simulink model "chap6_4sim"  (Simulink 3.00)
settings: Solver=ode45  StartTime=0.0  StopTime=3  RelTol=1e-3
settings Model: SaveTime=off  SaveOutput=off  Decimation=100  LastModifiedBy=liu

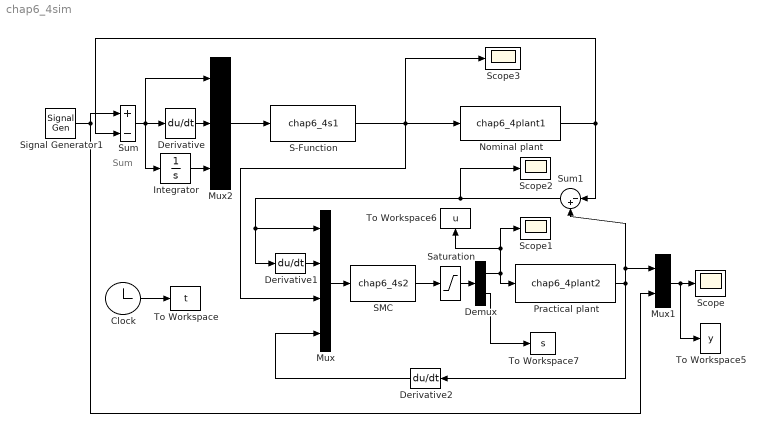
== system chap6_4sim ==
  note: Sum
  Clock : Clock
  Demux : Demux  Outputs=2
  Derivative : Derivative
  Derivative1 : Derivative
  Derivative2 : Derivative  Orientation=left
  Integrator : Integrator  ExternalReset=none  InitialConditionSource=internal  InitialCondition=0  LimitOutput=off  UpperSaturationLimit=inf  LowerSaturationLimit=-inf  ShowSaturationPort=off  ShowStatePort=off  AbsoluteTolerance=auto
  Mux : Mux  Inputs=4
      settings: DisplayOption=none
  Mux1 : Mux  Inputs=2
      settings: DisplayOption=none
  Mux2 : Mux  Inputs=3
      settings: DisplayOption=none
  Nominal plant : S-Function  FunctionName=chap6_4plant1  PortCounts=[]  SFunctionModules=''
  Practical plant : S-Function  FunctionName=chap6_4plant2  PortCounts=[]  SFunctionModules=''
  S-Function : S-Function  FunctionName=chap6_4s1  PortCounts=[]  SFunctionModules=''
  SMC : S-Function  FunctionName=chap6_4s2  PortCounts=[]  SFunctionModules=''
  Saturation : Saturate  UpperLimit=110  LowerLimit=-110
  Scope{,1..3} (4 alike) : Scope
      Scope settings: TimeRange=auto  YMin=-0.55  YMax=0.5  SaveToWorkspace=off  SaveName=ScopeData  MaxRows=50000
      Scope1 settings: TimeRange=auto  YMin=-5.5  YMax=3.5  SaveToWorkspace=off  SaveName=ScopeData
      Scope2 settings: TimeRange=auto  YMin=-0.00095  YMax=0.0001  SaveToWorkspace=off  SaveName=ScopeData  MaxRows=50000
      Scope3 settings: TimeRange=auto  YMin=0.2  YMax=2.3  SaveToWorkspace=off  SaveName=ScopeData  MaxRows=50000
  Signal Generator1 : SignalGenerator  WaveForm=sine  Amplitude=0.5  Frequency=3  Units=Hertz
  Sum : Sum  Inputs=|+-  SaturateOnIntegerOverflow=on
  Sum1 : Sum  Orientation=left  Inputs=|-+  SaturateOnIntegerOverflow=on
  To Workspace : ToWorkspace  VariableName=t  SampleTime=-1  SaveFormat=Matrix
  To Workspace5 : ToWorkspace  VariableName=y  SampleTime=-1  SaveFormat=Matrix
  To Workspace6 : ToWorkspace  VariableName=u  SampleTime=-1  SaveFormat=Matrix
      settings: Orientation=up
  To Workspace7 : ToWorkspace  VariableName=s  SampleTime=-1  SaveFormat=Matrix
  wires:
  Sum1/1 -> Mux/1, Derivative1/1, Scope2/1
  Derivative1/1 -> Mux/2
  Derivative2/1 -> Mux/4
  Demux/2 -> To Workspace7/1
  Demux/1 -> Practical plant/1, Scope1/1, To Workspace6/1
  Clock/1 -> To Workspace/1
  Mux/1 -> SMC/1
  Derivative/1 -> Mux2/2
  Sum/1 -> Derivative/1, Mux2/1, Integrator/1
  Integrator/1 -> Mux2/3
  SMC/1 -> Saturation/1
  Saturation/1 -> Demux/1
  Signal Generator1/1 -> Sum/1, Mux1/2
  Mux2/1 -> S-Function/1
  Mux1/1 -> Scope/1, To Workspace5/1
  Practical plant/1 -> Sum1/2, Mux1/1, Derivative2/1
  Nominal plant/1 -> Sum1/1, Sum/2
  S-Function/1 -> Scope3/1, Nominal plant/1, Mux/3
